simulink model "SOP_Estimator"  (R2022b)
settings: Solver=VariableStepAuto  StartTime=0.0  StopTime=10.0  RelTol=1e-3
values from neighbouring files (symbols this model uses):
  L_SOP = 10.0    [Estimators_Dictionary.sldd]
  MaxChargeCurrent = -4.5    [Estimators_Dictionary.sldd]
  MaxDischargeCurrent = 13.5    [Estimators_Dictionary.sldd]
  NumberSt = 4.0    [Estimators_Dictionary.sldd]
  NumModules = 1.0    [Global_Parameters.sldd]
  NumSeries = 24.0    [Global_Parameters.sldd]
  Ts_SOP = 15.0    [Estimators_Dictionary.sldd]
  Vmax = 4.1    [Global_Parameters.sldd]
  Vmin = 3.0    [Global_Parameters.sldd]
settings Model: DataDictionary=Estimators_Dictionary.sldd  Creator=japerez  LastModifiedBy=japerez

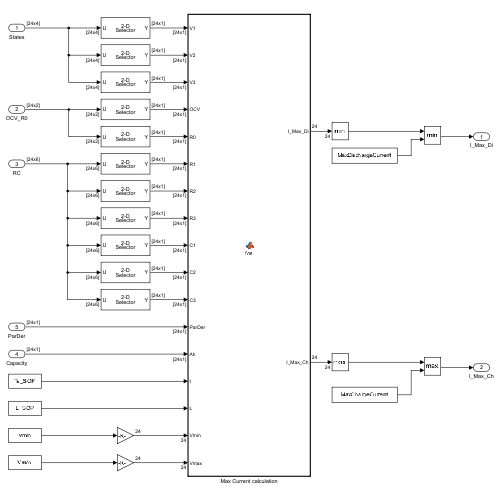
[thumbnail: Simulink's stored preview of the top-level diagram]
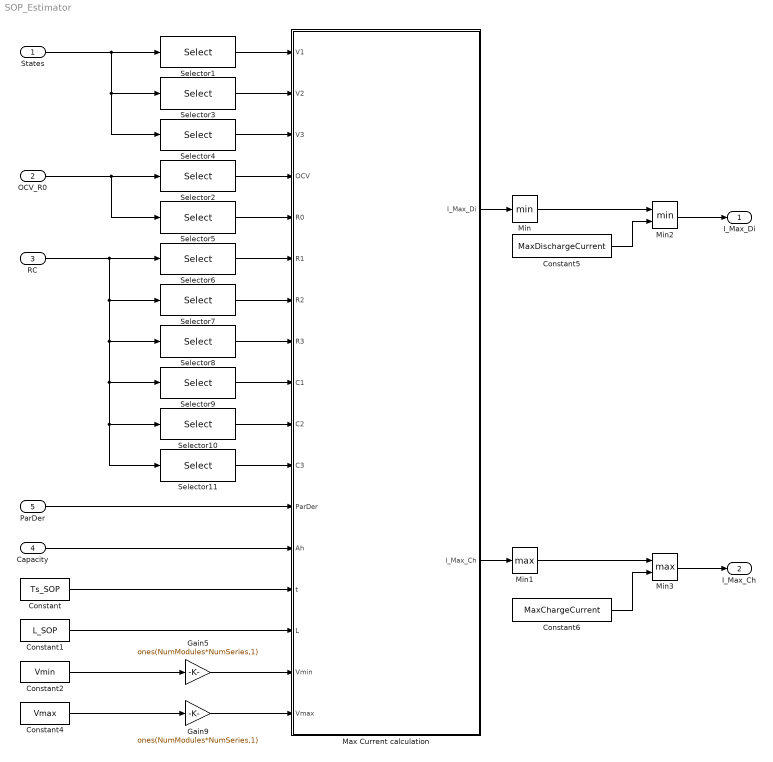
== system SOP_Estimator ==
  States : Inport  OutDataTypeStr=single  PortDimensions=[NumModules*NumSeries,NumberSt]
  OCV_R0 : Inport  Port=2  OutDataTypeStr=single  PortDimensions=[NumModules*NumSeries,2]
  RC : Inport  Port=3  OutDataTypeStr=single  PortDimensions=[NumModules*NumSeries,6]
  Capacity : Inport  Port=4  OutDataTypeStr=single  PortDimensions=[NumModules*NumSeries,1]
  ParDer : Inport  Port=5  OutDataTypeStr=single  PortDimensions=[NumModules*NumSeries,1]
  Constant : Constant  Value=Ts_SOP
  Constant1 : Constant  Value=L_SOP
  Constant2 : Constant  Value=Vmin  OutDataTypeStr=single
  Constant4 : Constant  Value=Vmax  OutDataTypeStr=single
  Constant5 : Constant  Value=MaxDischargeCurrent
  Constant6 : Constant  Value=MaxChargeCurrent
  Gain5 : Gain  Gain=ones(NumModules*NumSeries,1)  ParamDataTypeStr=single  OutDataTypeStr=single
  Gain9 : Gain  Gain=ones(NumModules*NumSeries,1)  ParamDataTypeStr=single  OutDataTypeStr=single
  Max Current calculation : MATLAB Function  TreatAsAtomicUnit=on
  Min : MinMax
  Min1 : MinMax  Function=max
  Min2 : MinMax  Inputs=2
  Min3 : MinMax  Function=max  Inputs=2
  Selector1 : Selector  NumberOfDimensions=2  InputPortWidth=24  IndexOptions=Select all,Index vector (dialog)  Indices=1,2  OutputSizes=1,1
  Selector10 : Selector  NumberOfDimensions=2  InputPortWidth=24  IndexOptions=Select all,Index vector (dialog)  Indices=1,5  OutputSizes=1,1
  Selector11 : Selector  NumberOfDimensions=2  InputPortWidth=24  IndexOptions=Select all,Index vector (dialog)  Indices=1,6  OutputSizes=1,1
  Selector2 : Selector  NumberOfDimensions=2  InputPortWidth=24  IndexOptions=Select all,Index vector (dialog)  Indices=1,1  OutputSizes=1,1
  Selector3 : Selector  NumberOfDimensions=2  InputPortWidth=24  IndexOptions=Select all,Index vector (dialog)  Indices=1,3  OutputSizes=1,1
  Selector4 : Selector  NumberOfDimensions=2  InputPortWidth=24  IndexOptions=Select all,Index vector (dialog)  Indices=1,4  OutputSizes=1,1
  Selector5 : Selector  NumberOfDimensions=2  InputPortWidth=24  IndexOptions=Select all,Index vector (dialog)  Indices=1,2  OutputSizes=1,1
  Selector6 : Selector  NumberOfDimensions=2  InputPortWidth=24  IndexOptions=Select all,Index vector (dialog)  Indices=1,1  OutputSizes=1,1
  Selector7 : Selector  NumberOfDimensions=2  InputPortWidth=24  IndexOptions=Select all,Index vector (dialog)  Indices=1,2  OutputSizes=1,1
  Selector8 : Selector  NumberOfDimensions=2  InputPortWidth=24  IndexOptions=Select all,Index vector (dialog)  Indices=1,3  OutputSizes=1,1
  Selector9 : Selector  NumberOfDimensions=2  InputPortWidth=24  IndexOptions=Select all,Index vector (dialog)  Indices=1,4  OutputSizes=1,1
  I_Max_Di : Outport  OutDataTypeStr=single  PortDimensions=1
  I_Max_Ch : Outport  Port=2  OutDataTypeStr=single  PortDimensions=1
  wires:
  Constant2/1 -> Gain5/1
  Constant4/1 -> Gain9/1
  Gain5/1 -> Max Current calculation/16(Vmin)
  Gain9/1 -> Max Current calculation/17(Vmax)
  Max Current calculation/1(I_Max_Di) -> Min/1
  Min2/1 -> I_Max_Di/1
  Min3/1 -> I_Max_Ch/1
  Max Current calculation/2(I_Max_Ch) -> Min1/1
  Constant/1 -> Max Current calculation/14(t)
  Constant1/1 -> Max Current calculation/15(L)
  Constant5/1 -> Min2/2
  Constant6/1 -> Min3/2
  Min/1 -> Min2/1
  Min1/1 -> Min3/1
  Selector3/1 -> Max Current calculation/2(V2)
  Selector1/1 -> Max Current calculation/1(V1)
  Selector4/1 -> Max Current calculation/3(V3)
  States/1 -> Selector4/1, Selector3/1, Selector1/1
  Selector2/1 -> Max Current calculation/4(OCV)
  Selector5/1 -> Max Current calculation/5(R0)
  OCV_R0/1 -> Selector5/1, Selector2/1
  Selector6/1 -> Max Current calculation/6(R1)
  Selector7/1 -> Max Current calculation/7(R2)
  Selector8/1 -> Max Current calculation/8(R3)
  Selector9/1 -> Max Current calculation/9(C1)
  Selector10/1 -> Max Current calculation/10(C2)
  Selector11/1 -> Max Current calculation/11(C3)
  RC/1 -> Selector11/1, Selector10/1, Selector9/1, Selector8/1, Selector7/1, Selector6/1
  ParDer/1 -> Max Current calculation/12(ParDer)
  Capacity/1 -> Max Current calculation/13(Ah)

== matlab function SOP_Estimator/Max Current calculation ==
  data: V1 input; V2 input; V3 input; OCV input single; R0 input single; R1 input single; R2 input single; R3 input single; C1 input single; C2 input single; C3 input single; ParDer input; Ah input single; I_Max_Di output single; t input; L input; Vmin input; Vmax input; I_Max_Ch output single
function [I_Max_Di,I_Max_Ch] = fcn(V1,V2,V3,OCV,R0,R1,R2,R3,C1,C2,C3,ParDer,Ah,t,L,Vmin,Vmax)

% Temporal constants
tau1=R1.*C1;
tau2=R2.*C2;
tau3=R3.*C3;
% Equations
Numerator= OCV-V1.*exp((-L*t)./tau1)-V2.*exp((-L*t)./tau2)-V3.*exp((-L*t)./tau3);
Denominator= ((L*t./(Ah*3600)).*ParDer)+R0+R1.*(1-exp((-L*t)./tau1))+R2.*(1-exp((-L*t)./tau2))+R3.*(1-exp((-L*t)./tau3));

I_Max_Di = (Numerator-Vmin)./Denominator;

I_Max_Ch = (Numerator-Vmax)./Denominator;
